simulink model "generic_20231123_1032"  (R2022b)
settings: Solver=ode45  StartTime=0.0  StopTime=50  RelTol=1e-3  EnableMultiTasking=on
model workspace (MAT data in the model file):
  A = 1
  Amplifier = -9.10007585438
  B = 1.19071237887
  K_d_yawrate = 0.231634180251
  K_dsteering = 5.24463953925
  k_speed = -0.570636497542
  k_stanley = 28.4909595466
  kd = -9.99955278144
  ki = 0.00519416981022
  kp = 9.99999979837
  path_curvature = 0
values from neighbouring files (symbols this model uses):
  brake_select = ones(length(speed), length(steering_angle))    [TwoDLook_uptable.m]
  curvature = 0.000:0.001:1    [TwoDLook_uptable.m]
  m = 1600    [MPCController1.m]    (also in MPCController2.m; MPC_Fmincon.m)
  speed = 0:0.1:100    [TwoDLook_uptable.m]
  steering_angle = -3.14/4:0.00628/4:3.14/4    [TwoDLook_uptable.m]
undefined symbols (not defined in the file or in its folder): DiscIntNeverNeededParam
libraries: CarMaker4SL x143, simulink x11, cstblocks x6, simulink_extras x4, autolibshared x1, mpcadaslib x1
(part 2 of 7)

== system generic_20231123_1032/CarMaker/IPG Vehicle/CarAndTrailer/Kinematics ==
  Sync_In : Inport
  Steer.IF : Inport  Port=2
  Kinematics : S-Function  FunctionName=CM_Sfun  Parameters='Kinematics'  SFunctionDeploymentMode=off  EnableBusSupport=off
  Sync_Out : Outport  VectorParamsAs1DForOutWhenUnconnected=off
  TireFL_In : Outport  Port=2  VectorParamsAs1DForOutWhenUnconnected=off
  TireFR_In : Outport  Port=3  VectorParamsAs1DForOutWhenUnconnected=off
  TireRL_In : Outport  Port=4  VectorParamsAs1DForOutWhenUnconnected=off
  TireRR_In : Outport  Port=5  VectorParamsAs1DForOutWhenUnconnected=off
  lSpring : Outport  Port=6  VectorParamsAs1DForOutWhenUnconnected=off
  vDamp : Outport  Port=7  VectorParamsAs1DForOutWhenUnconnected=off
  lStabi : Outport  Port=8  VectorParamsAs1DForOutWhenUnconnected=off
  lBuf : Outport  Port=9  VectorParamsAs1DForOutWhenUnconnected=off
  wires:
  Kinematics/9 -> lBuf/1
  Kinematics/8 -> lStabi/1
  Kinematics/2 -> TireFL_In/1
  Kinematics/3 -> TireFR_In/1
  Kinematics/4 -> TireRL_In/1
  Kinematics/5 -> TireRR_In/1
  Kinematics/6 -> lSpring/1
  Kinematics/7 -> vDamp/1
  Sync_In/1 -> Kinematics/1
  Kinematics/1 -> Sync_Out/1
  Steer.IF/1 -> Kinematics/2

== system generic_20231123_1032/CarMaker/IPG Vehicle/CarAndTrailer/Kinetics ==
  Sync_In : Inport
  Car.Virtual : Inport  Port=2
  Car.Aero : Inport  Port=3
  Car.Load : Inport  Port=4
  TireFL.Out : Inport  Port=5
  TireFR.Out : Inport  Port=6
  TireRL.Out : Inport  Port=7
  TireRR.Out : Inport  Port=8
  FSpring_ext : Inport  Port=9
  FDamp_ext : Inport  Port=10
  FStabi_ext : Inport  Port=11
  FBuf_ext : Inport  Port=12
  Bus Creator : BusCreator  Inputs=4
  Bus Creator1 : BusCreator  Inputs=12
  Bus Creator2 : BusCreator  Inputs=6
  Bus Creator3 : BusCreator  Inputs=6
  Bus Creator4 : BusCreator  Inputs=4
  Demux : Demux  Outputs=12
      settings: DisplayOption=none
  Demux1 : Demux  Outputs=6
      settings: DisplayOption=none
  Demux2 : Demux  Outputs=6
      settings: DisplayOption=none
  Demux3 : Demux
      settings: DisplayOption=none
  Demux4 : Demux
      settings: DisplayOption=none
  Kinetics : S-Function  FunctionName=CM_Sfun  Parameters='Kinetics'  SFunctionDeploymentMode=off  EnableBusSupport=off
  Sync_Out : Outport  VectorParamsAs1DForOutWhenUnconnected=off
  Trailer.Load : Outport  Port=2  VectorParamsAs1DForOutWhenUnconnected=off
  Car.Hitch : Outport  Port=3  VectorParamsAs1DForOutWhenUnconnected=off
  Car.Fr1 : Outport  Port=4  VectorParamsAs1DForOutWhenUnconnected=off
  Car.Trq_T2W : Outport  Port=5  VectorParamsAs1DForOutWhenUnconnected=off
  WheelCarrier.Misc : Outport  Port=6  VectorParamsAs1DForOutWhenUnconnected=off
  wires:
  FBuf_ext/1 -> Kinetics/12
  Sync_In/1 -> Kinetics/1
  Kinetics/1 -> Sync_Out/1
  Car.Aero/1 -> Kinetics/3
  Car.Virtual/1 -> Kinetics/2
  Bus Creator1/1 -> Trailer.Load/1
  Demux/1 -> Bus Creator1/1  "Trailer Load_0 mass"
  Demux/2 -> Bus Creator1/2  "Trailer Load_0 tx"
  Demux/3 -> Bus Creator1/3  "Trailer Load_0 ty"
  Demux/4 -> Bus Creator1/4  "Trailer Load_0 tz"
  Kinetics/2 -> Demux/1
  Demux/5 -> Bus Creator1/5  "Trailer Load_1 mass"
  Demux/6 -> Bus Creator1/6  "Trailer Load_1 tx"
  Demux/7 -> Bus Creator1/7  "Trailer Load_1 ty"
  Demux/8 -> Bus Creator1/8  "Trailer Load_1 tz"
  Demux/9 -> Bus Creator1/9  "Trailer Load_2 mass"
  Demux/10 -> Bus Creator1/10  "Trailer Load_2 tx"
  Demux/11 -> Bus Creator1/11  "Trailer Load_2 ty"
  Demux/12 -> Bus Creator1/12  "Trailer Load_2 tz"
  Demux1/1 -> Bus Creator2/1  "Car Hitch tx"
  Demux1/2 -> Bus Creator2/2  "Car Hitch ty"
  Demux1/3 -> Bus Creator2/3  "Car Hitch tz"
  Demux1/4 -> Bus Creator2/4  "Car Hitch vx"
  Demux1/5 -> Bus Creator2/5  "Car Hitch vy"
  Demux1/6 -> Bus Creator2/6  "Car Hitch vz"
  Kinetics/3 -> Demux1/1
  Bus Creator2/1 -> Car.Hitch/1
  Demux2/1 -> Bus Creator3/1  "Car Fr1 rx"
  Demux2/2 -> Bus Creator3/2  "Car Fr1 ry"
  Demux2/3 -> Bus Creator3/3  "Car Fr1 rz"
  Demux2/4 -> Bus Creator3/4  "Car Fr1 rvx"
  Demux2/5 -> Bus Creator3/5  "Car Fr1 rvy"
  Demux2/6 -> Bus Creator3/6  "Car Fr1 rvz"
  Bus Creator3/1 -> Car.Fr1/1
  Kinetics/4 -> Demux2/1
  Car.Load/1 -> Kinetics/4
  Demux3/1 -> Bus Creator4/1  "car Susp FL GenInert2"
  Demux3/2 -> Bus Creator4/2  "car Susp FR GenInert2"
  Demux3/3 -> Bus Creator4/3  "car Susp FL GenFrc2"
  Demux3/4 -> Bus Creator4/4  "car Susp FR GenFrc2"
  Bus Creator4/1 -> WheelCarrier.Misc/1
  Bus Creator/1 -> Car.Trq_T2W/1
  Demux4/4 -> Bus Creator/4  "Car Trq_T2WRR"
  Demux4/3 -> Bus Creator/3  "Car Trq_T2WRL"
  Demux4/2 -> Bus Creator/2  "Car Trq_T2WFR"
  Demux4/1 -> Bus Creator/1  "Car Trq_T2WFL"
  TireFL.Out/1 -> Kinetics/5
  TireFR.Out/1 -> Kinetics/6
  TireRL.Out/1 -> Kinetics/7
  TireRR.Out/1 -> Kinetics/8
  FSpring_ext/1 -> Kinetics/9
  FDamp_ext/1 -> Kinetics/10
  FStabi_ext/1 -> Kinetics/11
  Kinetics/6 -> Demux3/1
  Kinetics/5 -> Demux4/1

== system generic_20231123_1032/CarMaker/IPG Vehicle/CarAndTrailer/Steering ==
  note: When replacing the entire steering system,
      | be sure to disable the IPG steering model by using the steering
      | model 'Model Manager off' in the vehicle GUI.
  Sync_In : Inport
  VhclCtrl.Steering : Inport  Port=2
  Bus Creator1 : BusCreator  Inputs=16
  Bus Creator2 : BusCreator  Inputs=5
  Demux : Demux  Outputs=21
      settings: DisplayOption=none
  Steering : S-Function  FunctionName=CM_Sfun  Parameters='Steering'  SFunctionDeploymentMode=off  EnableBusSupport=off
  Terminator : Terminator
  Sync_Out : Outport  VectorParamsAs1DForOutWhenUnconnected=off
  Steer.IF : Outport  Port=2  VectorParamsAs1DForOutWhenUnconnected=off
  wires:
  Demux/21 -> Bus Creator2/5  "Steering IF R Inert"
  Demux/20 -> Bus Creator2/4  "Steering IF R Frc"
  Demux/19 -> Bus Creator2/3  "Steering IF L Inert"
  Demux/18 -> Bus Creator2/2  "Steering IF L Frc"
  Demux/17 -> Bus Creator2/1  "Steering IF SteerByTrq"
  Demux/16 -> Bus Creator1/16  "Steering IF R iSteer2q"
  Demux/15 -> Bus Creator1/15  "Steering IF R qpp"
  Demux/14 -> Bus Creator1/14  "Steering IF R qp"
  Demux/13 -> Bus Creator1/13  "Steering IF R q"
  Demux/12 -> Bus Creator1/12  "Steering IF L iSteer2q"
  Demux/11 -> Bus Creator1/11  "Steering IF L qpp"
  Demux/10 -> Bus Creator1/10  "Steering IF L qp"
  Demux/9 -> Bus Creator1/9  "Steering IF L q"
  Demux/8 -> Bus Creator1/8  "Steering IF AssistTrqPin"
  Demux/7 -> Bus Creator1/7  "Steering IF AssistTrqCol"
  Demux/6 -> Bus Creator1/6  "Steering IF AssistFrc"
  Demux/5 -> Bus Creator1/5  "Steering IF TrqStatic"
  Demux/4 -> Bus Creator1/4  "Steering IF Trq"
  Demux/3 -> Bus Creator1/3  "Steering IF AngAcc"
  Demux/2 -> Bus Creator1/2  "Steering IF AngVel"
  Demux/1 -> Bus Creator1/1  "Steering IF Ang"
  Bus Creator1/1 -> Steer.IF/1
  Steering/2 -> Demux/1
  Bus Creator2/1 -> Terminator/1  "Steer IF (in)"
  VhclCtrl.Steering/1 -> Steering/2
  Steering/1 -> Sync_Out/1
  Sync_In/1 -> Steering/1

== system generic_20231123_1032/CarMaker/IPG Vehicle/CarAndTrailer/Trailer ==
  Sync_In : Inport
  Trailer.Load : Inport  Port=2
  Car.Hitch : Inport  Port=3
  Car.Fr1 : Inport  Port=4
  Car.Trq_T2W : Inport  Port=5
  WheelCarrier.Misc : Inport  Port=6
  CreateBus Car.Hitch.FrcTrq : Subsystem
  CreateBus Vhcl.Motion : Subsystem
  CreateBus Vhcl.PoI : Subsystem
  CreateBus Vhcl.Steering : Subsystem
  CreateBus Vhcl.Wheel.FL : Subsystem
  CreateBus Vhcl.Wheel.FR : Subsystem
  CreateBus Vhcl.Wheel.RL : Subsystem
  CreateBus Vhcl.Wheel.RR : Subsystem
  Trailer : S-Function  FunctionName=CM_Sfun  Parameters='Trailer'  SFunctionDeploymentMode=off  EnableBusSupport=off
  Sync_Out : Outport  VectorParamsAs1DForOutWhenUnconnected=off
  Vhcl.Steering : Outport  Port=2  VectorParamsAs1DForOutWhenUnconnected=off
  Vhcl.Motion : Outport  Port=3  VectorParamsAs1DForOutWhenUnconnected=off
  Vhcl.PoI : Outport  Port=4  VectorParamsAs1DForOutWhenUnconnected=off
  Vhcl.Wheel.FL : Outport  Port=5  VectorParamsAs1DForOutWhenUnconnected=off
  Vhcl.Wheel.FR : Outport  Port=6  VectorParamsAs1DForOutWhenUnconnected=off
  Vhcl.Wheel.RL : Outport  Port=7  VectorParamsAs1DForOutWhenUnconnected=off
  Vhcl.Wheel.RR : Outport  Port=8  VectorParamsAs1DForOutWhenUnconnected=off
  Car.Hitch.FrcTrq : Outport  Port=9  VectorParamsAs1DForOutWhenUnconnected=off
  wires:
  Trailer/2 -> CreateBus Vhcl.Steering/1(In1)
  CreateBus Vhcl.Steering/1(Out1) -> Vhcl.Steering/1  "Vhcl.Steering"
  Trailer/3 -> CreateBus Vhcl.Motion/1(In1)
  Trailer/4 -> CreateBus Vhcl.PoI/1(In1)
  Trailer/5 -> CreateBus Vhcl.Wheel.FL/1(In1)
  Trailer/6 -> CreateBus Vhcl.Wheel.FR/1(In1)
  Trailer/7 -> CreateBus Vhcl.Wheel.RL/1(In1)
  Trailer/9 -> CreateBus Car.Hitch.FrcTrq/1(In1)
  Trailer/8 -> CreateBus Vhcl.Wheel.RR/1(In1)
  CreateBus Vhcl.Wheel.RR/1(Out1) -> Vhcl.Wheel.RR/1  "Vhcl.Wheel.RR"
  CreateBus Vhcl.Wheel.RL/1(Out1) -> Vhcl.Wheel.RL/1  "Vhcl.Wheel.RL"
  CreateBus Vhcl.Wheel.FR/1(Out1) -> Vhcl.Wheel.FR/1  "Vhcl.Wheel.FR"
  CreateBus Vhcl.Wheel.FL/1(Out1) -> Vhcl.Wheel.FL/1  "Vhcl.Wheel.FL"
  CreateBus Vhcl.PoI/1(Out1) -> Vhcl.PoI/1  "Vhcl.PoI"
  CreateBus Vhcl.Motion/1(Out1) -> Vhcl.Motion/1  "Vhcl.Motion"
  Car.Trq_T2W/1 -> Trailer/5
  WheelCarrier.Misc/1 -> Trailer/6
  CreateBus Car.Hitch.FrcTrq/1(Out1) -> Car.Hitch.FrcTrq/1  "Car.Hitch.FrcTrq"
  Car.Fr1/1 -> Trailer/4
  Car.Hitch/1 -> Trailer/3
  Trailer.Load/1 -> Trailer/2
  Trailer/1 -> Sync_Out/1
  Sync_In/1 -> Trailer/1

== system generic_20231123_1032/CarMaker/VehicleControl/CreateBus VhclCtrl/A*algoithm ==
  Bus Selector1 : BusSelector  OutputSignals=Path.tx,Path.ty
  Constant : Constant  Value=0
  Constant3 : Constant  Value=0
  Constant4 : Constant
  Gain : Gain  Gain=2
  MATLAB Function1 : MATLAB Function  TreatAsAtomicUnit=on
  Mux : Mux  Inputs=2
  Mux1 : Mux  Inputs=2
  Mux2 : Mux  Inputs=2
  Read CM Dict3 : CarMaker4SL/Read CM Dict  xname=Sensor.Radar.VehSensor_6.Obj0.Length  xsync=off  xstime=Continuous
  Read CM Dict4 : CarMaker4SL/Read CM Dict  xname=Traffic.T00.tx  xsync=off  xstime=Continuous
  Read CM Dict5 : CarMaker4SL/Read CM Dict  xname=Traffic.T00.ty  xsync=off  xstime=Continuous
  Read CM Dict6 : CarMaker4SL/Read CM Dict  xname=Sensor.Radar.VehSensor_6.Obj0.ProbObst  xsync=off  xstime=Continuous
  Read CM Dict7 : CarMaker4SL/Read CM Dict  xname=Sensor.Radar.VehSensor_6.Obj0.Width  xsync=off  xstime=Continuous
  Reshape : Reshape  OutputDimensionality=Customize  OutputDimensions=[1,2]
  Reshape1 : Reshape  OutputDimensionality=Customize  OutputDimensions=[1,2]
  Reshape2 : Reshape  OutputDimensionality=Customize  OutputDimensions=[1,2]
  Road Sensor1 : CarMaker4SL/Sensors/Road Sensor  xname=0  xstime=Continuous
      settings: SourceProductName=CarMaker4SL
  Subsystem : Subsystem  Commented=on
  Sum : Sum  Inputs=|++
  Switch : Switch  Criteria=u2 > Threshold  SaturateOnIntegerOverflow=off  InputSameDT=off
  Terminator : Terminator
  Terminator1 : Terminator
  Terminator2 : Terminator
  deviation : Outport
  pathX : Outport  Port=2
  pathY : Outport  Port=3
  wires:
  Constant4/1 -> Switch/1
  Road Sensor1/2 -> Bus Selector1/1
  Road Sensor1/1 -> Terminator/1
  Read CM Dict4/1 -> Mux1/1, Mux/1
  Constant3/1 -> Road Sensor1/1
  Read CM Dict6/1 -> Switch/2
  Constant/1 -> Switch/3
  Read CM Dict3/1 -> Gain/1
  Gain/1 -> Sum/1
  Read CM Dict5/1 -> Sum/2, Mux/2
  Mux2/1 -> Reshape/1
  Bus Selector1/1 -> Mux2/1  "<tx>"
  Bus Selector1/2 -> Mux2/2  "<ty>"
  Sum/1 -> Mux1/2
  Mux1/1 -> Reshape1/1
  Mux/1 -> Reshape2/1
  Reshape/1 -> MATLAB Function1/1(start)
  Reshape1/1 -> MATLAB Function1/2(target)
  Reshape2/1 -> MATLAB Function1/3(obstacles)
  MATLAB Function1/1(deviation) -> deviation/1
  MATLAB Function1/2(pathX) -> pathX/1
  MATLAB Function1/3(pathY) -> pathY/1
  Switch/1 -> Terminator1/1
  Read CM Dict7/1 -> Terminator2/1

== system generic_20231123_1032/CarMaker/VehicleControl/CreateBus VhclCtrl/MPC_steering_controllers ==
  Lateral_dev : Inport
  Dev_angle : Inport  Port=2
  Amplifyer : Gain  Gain=Amplifier
  Amplifyer1 : Gain  Gain=2
  Amplifyer2 : Gain  Gain=-3
  Bus Selector1 : BusSelector  OutputSignals=Path.tx,Path.ty,Path,Path.DevAng,Path.CurveXY
  Constant1 : Constant  Value=3
  Constant2 : Constant  Value=0
  Demux : Demux  Outputs=5
  Discrete-Time Integrator : DiscreteIntegrator  SampleTime=-1  ICPrevOutput=DiscIntNeverNeededParam  ICPrevScaledInput=DiscIntNeverNeededParam
  Gain : Gain  Gain=-1.6
  MATLAB System : MATLABSystem  Commented=on  System=MPCController  Nx=5  Nu=1  Ny=2  Np=20  Nc=10  T=0.01  lf=1.488  lr=1.487  Ccf=66900  Ccr=62700  m=1600  g=9.81  I=2986.624  x_dot=15  Q=diag( [ 2000, 0, 0, 10000, 0 ] )  R=5 * 10 ^ 5  Row=1000  umin=-0.6  umax=0.6  delta_umin=-0.06  delta_umax=0.06  ycmax=[ 0.2; 1000 ]  ycmin=[ -0.2; -1000 ]  SimulateUsing=Code generation
      mask Type: MPCController
      mask Display:
      | disp('MPCController');
      | port_label('input',1,'y_dot');
      | port_label('input',2,'phi');
      | port_label('input',3,'phi_dot');
      | port_label('input',4,'Y');
      | port_label('input',5,'X');
      | port_label('output',1,'delta_f');
      | port_label('output',2,'state_k1');
  Multiport Switch : MultiPortSwitch  SaturateOnIntegerOverflow=off  InputSameDT=off
  Mux1 : Mux  Inputs=5
  Mux3 : Mux  Inputs=1
  Product : Product
  Radians to Degrees : simulink_extras/Transformations/Radians to Degrees
  Radians to Degrees1 : simulink_extras/Transformations/Radians to Degrees
  Read CM Dict : CarMaker4SL/Read CM Dict  xname=Sensor.Road.VehSensor_0.Path.DevAng  xsync=off  xstime=Continuous
  Read CM Dict1 : CarMaker4SL/Read CM Dict  xname=Car.Road.Path.DevDist  xsync=off  xstime=Continuous
  Read CM Dict8 : CarMaker4SL/Read CM Dict  xname=Vhcl.v  xsync=off  xstime=Continuous
  Road Sensor1 : CarMaker4SL/Sensors/Road Sensor  xname=0  xstime=Continuous
      settings: SourceProductName=CarMaker4SL
  S-Function1 : S-Function  FunctionName=MPCController1  SFunctionDeploymentMode=off  EnableBusSupport=off
  Scope : Scope
  Sign : Signum
  State_space_system_variables : Subsystem
  Subsystem : Subsystem  Commented=on
  Sum : Sum  Inputs=|+++
  Terminator : Terminator
  Terminator1 : Terminator  Commented=on
  Terminator2 : Terminator
  Terminator3 : Terminator
  Traditional_MPC : Subsystem
  steering : Outport
  wires:
  Constant2/1 -> Road Sensor1/1
  Demux/1 -> MATLAB System/4
  Bus Selector1/5 -> Product/2  "<CurveXY>"
  Bus Selector1/3 -> Terminator1/1  "<Path>"
  Road Sensor1/1 -> Terminator/1
  Road Sensor1/2 -> Bus Selector1/1
  Mux3/1 -> S-Function1/1, Demux/1
  Read CM Dict8/1 -> Product/1
  Bus Selector1/1 -> State_space_system_variables/3(X_ref_m), Mux1/5  "<tx>"
  Bus Selector1/2 -> State_space_system_variables/2(Y_ref_m), Mux1/4  "<ty>"
  Product/1 -> Discrete-Time Integrator/1, Radians to Degrees1/1
  Discrete-Time Integrator/1 -> Radians to Degrees/1
  Radians to Degrees/1 -> State_space_system_variables/1(Yaw_ref_deg), Mux1/2
  Constant1/1 -> Multiport Switch/1
  Radians to Degrees1/1 -> Mux1/3
  State_space_system_variables/1(x) -> Mux3/1
  Demux/5 -> MATLAB System/3
  Demux/3 -> MATLAB System/1
  State_space_system_variables/2(Lateral_velocity) -> Mux1/1
  Read CM Dict/1 -> Amplifyer/1
  Mux1/1 -> Terminator2/1  "u"
  Read CM Dict1/1 -> Amplifyer1/1
  Amplifyer/1 -> Amplifyer2/1  "Dev_angle"
  Demux/2 -> MATLAB System/5
  Demux/4 -> MATLAB System/2
  Amplifyer1/1 -> Traditional_MPC/1(Lateral_deviation)  "Dev_angle"
  Amplifyer2/1 -> Traditional_MPC/2(Dev_angle)  "Dev_angle"
  MATLAB System/1 -> Multiport Switch/3
  Multiport Switch/1 -> steering/1
  MATLAB System/2 -> Terminator3/1
  S-Function1/1 -> Sign/1, Sum/1, Multiport Switch/2
  Traditional_MPC/1(steering_cmd) -> Multiport Switch/4
  Sum/1 -> Scope/1
  Traditional_MPC/2(Heading_correction) -> Sum/2
  Sign/1 -> Gain/1
  Gain/1 -> Sum/3

== system generic_20231123_1032/CarMaker/VehicleControl/CreateBus VhclCtrl/PID steering controller ==
  Lateral_error : Inport
  Add : Sum  Inputs=+++
  Dervative : Subsystem
  Discrete-Time Integrator : DiscreteIntegrator  SampleTime=-1  ICPrevOutput=DiscIntNeverNeededParam  ICPrevScaledInput=DiscIntNeverNeededParam
  Gain : Gain  Gain=1.1
  Gain1 : Gain  Gain=0.9
  steering_cmd : Outport
  wires:
  Lateral_error/1 -> Gain1/1, Gain/1, Dervative/1(Error)
  Discrete-Time Integrator/1 -> Add/1
  Gain1/1 -> Discrete-Time Integrator/1
  Gain/1 -> Add/2
  Add/1 -> steering_cmd/1
  Dervative/1(Dervative term) -> Add/3

== system generic_20231123_1032/CarMaker/VehicleControl/CreateBus VhclCtrl/Smoothing ==
  Signal_In : Inport
  Add : Sum  Inputs=++++
  Delay : Delay  InitialCondition=0.1
  Delay1 : Delay  DelayLength=4  InitialCondition=0.1
  Delay2 : Delay  DelayLength=5  InitialCondition=0.1
  Gain : Gain  Gain=0.35
  Gain1 : Gain  Gain=0.25
  Gain2 : Gain  Gain=0.25
  Gain3 : Gain  Gain=0.15
  Signal_Out : Outport  VectorParamsAs1DForOutWhenUnconnected=off
  wires:
  Gain1/1 -> Add/2
  Signal_In/1 -> Gain/1
  Delay/1 -> Gain1/1
  Gain/1 -> Add/1
  Delay1/1 -> Gain2/1
  Add/1 -> Delay2/1, Delay1/1, Delay/1, Signal_Out/1
  Gain2/1 -> Add/3
  Delay2/1 -> Gain3/1
  Gain3/1 -> Add/4

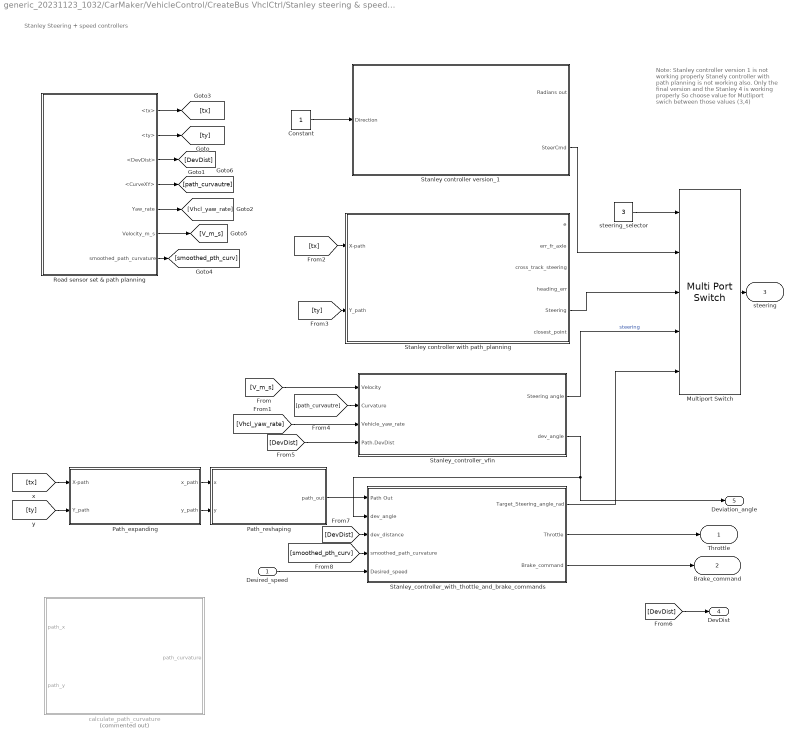
== system generic_20231123_1032/CarMaker/VehicleControl/CreateBus VhclCtrl/Stanley steering & speed//Brake controller ==
  note: Note:
      | Stanley controller version 1 is not working properly
      | Stanely controller with path planning is not working also.
      | Only the final version and the Stanley 4 is working properly
      | So choose value for Mutliport swich between those values (3,4)
  note: Stanley Steering + speed controllers
  Desired_speed : Inport
  " Path_expanding" : Subsystem
  Constant : Constant
  Multiport Switch : MultiPortSwitch  Inputs=4  SaturateOnIntegerOverflow=off  InputSameDT=off
  Path_reshaping : MATLAB Function  TreatAsAtomicUnit=on
  Road sensor set & path planning : Subsystem  Variant=on  VariantControlMode=label  VariantControl=Choice  LabelModeActiveChoice=Choice
  Stanley controller version_1 : Subsystem  Variant=on  VariantControlMode=label  VariantControl=Choice  LabelModeActiveChoice=Choice
  Stanley controller with path_planning : Subsystem  Variant=on  VariantControlMode=label  VariantControl=Choice  LabelModeActiveChoice=Choice
  Stanley_controller_vfin : Subsystem  Variant=on  VariantControlMode=label  VariantControl=Choice  LabelModeActiveChoice=Choice
  Stanley_controller_with_thottle_and_brake_commands : Subsystem
  calculate_path_curvature : Subsystem  Commented=on  Variant=on  VariantControlMode=label  VariantControl=Choice  LabelModeActiveChoice=Choice
  steering_selector : Constant  Value=3
  Throttle : Outport
  Brake_command : Outport  Port=2
  steering : Outport  Port=3
  DevDist : Outport  Port=4
  Deviation_angle : Outport  Port=5
  wires:
  [tx] -> " Path_expanding"/1(X-path)
  [ty] -> " Path_expanding"/2(Y_path)
  [tx] -> Stanley controller with path_planning/1(X-path)
  [ty] -> Stanley controller with path_planning/2(Y_path)
  Road sensor set & path planning/1(<tx>) -> [tx]
  Road sensor set & path planning/2(<ty>) -> [ty]
  Road sensor set & path planning/3(<DevDist>) -> [DevDist]
  Road sensor set & path planning/4(<CurveXY>) -> [path_curvautre]
  Road sensor set & path planning/5(Yaw_rate) -> [Vhcl_yaw_rate]
  [path_curvautre] -> Stanley_controller_vfin/2(Curvature)
  Stanley_controller_vfin/1(Steering angle) -> Multiport Switch/4  "steering"
  Constant/1 -> Stanley controller version_1/1(Direction)
  steering_selector/1 -> Multiport Switch/1
  Stanley controller version_1/2(SteerCmd) -> Multiport Switch/2
  Stanley controller with path_planning/5(Steering) -> Multiport Switch/3
  Path_reshaping/1(path_out) -> Stanley_controller_with_thottle_and_brake_commands/1(Path Out)
  Stanley_controller_vfin/2(dev_angle) -> Deviation_angle/1, Stanley_controller_with_thottle_and_brake_commands/2(dev_angle)
  " Path_expanding"/1(x_path) -> Path_reshaping/1(x)
  " Path_expanding"/2(y_path) -> Path_reshaping/2(y)
  Stanley_controller_with_thottle_and_brake_commands/2(Throttle) -> Throttle/1
  Stanley_controller_with_thottle_and_brake_commands/3(Brake_command) -> Brake_command/1
  Stanley_controller_with_thottle_and_brake_commands/1(Target_Steering_angle_rad) -> Multiport Switch/5
  [V_m_s] -> Stanley_controller_vfin/1(Velocity)
  [Vhcl_yaw_rate] -> Stanley_controller_vfin/3(Vehicle_yaw_rate)
  [DevDist] -> Stanley_controller_vfin/4(Path.DevDist)
  Road sensor set & path planning/6(Velocity_m_s) -> [V_m_s]
  [DevDist] -> DevDist/1
  Multiport Switch/1 -> steering/1
  [DevDist] -> Stanley_controller_with_thottle_and_brake_commands/3(dev_distance)
  Road sensor set & path planning/7(smoothed_path_curvature) -> [smoothed_pth_curv]
  [smoothed_pth_curv] -> Stanley_controller_with_thottle_and_brake_commands/4(smoothed_path_curvature)
  Desired_speed/1 -> Stanley_controller_with_thottle_and_brake_commands/5(Desired_speed)

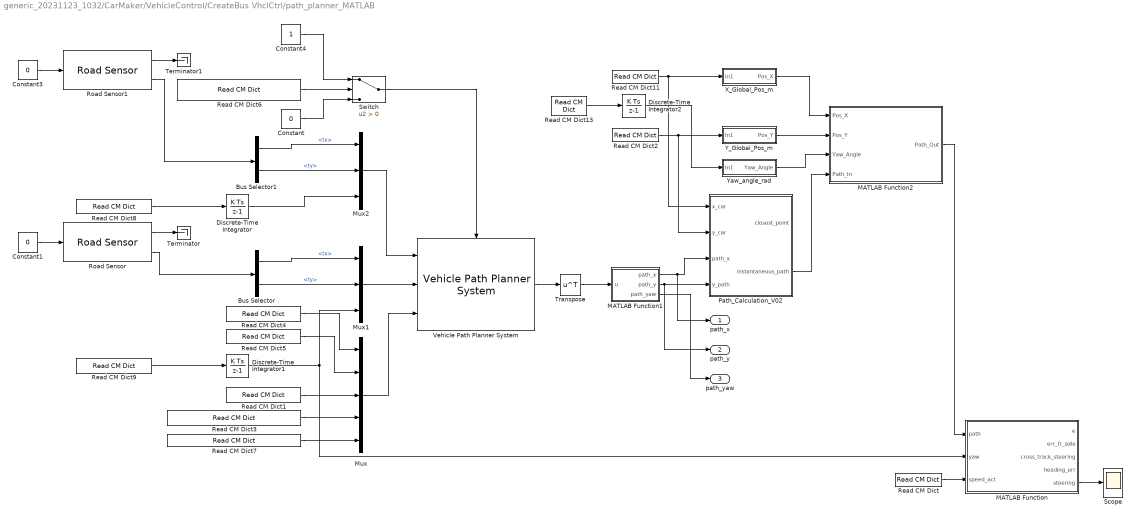
== system generic_20231123_1032/CarMaker/VehicleControl/CreateBus VhclCtrl/path_planner_MATLAB ==
  Bus Selector : BusSelector  OutputSignals=Path.tx,Path.ty
  Bus Selector1 : BusSelector  OutputSignals=Path.tx,Path.ty
  Constant : Constant  Value=0
  Constant1 : Constant  Value=0
  Constant3 : Constant  Value=0
  Constant4 : Constant
  Discrete-Time Integrator : DiscreteIntegrator  SampleTime=-1  ICPrevOutput=DiscIntNeverNeededParam  ICPrevScaledInput=DiscIntNeverNeededParam
  Discrete-Time Integrator1 : DiscreteIntegrator  SampleTime=-1  ICPrevOutput=DiscIntNeverNeededParam  ICPrevScaledInput=DiscIntNeverNeededParam
  Discrete-Time Integrator2 : DiscreteIntegrator  SampleTime=-1  ICPrevOutput=DiscIntNeverNeededParam  ICPrevScaledInput=DiscIntNeverNeededParam
  MATLAB Function : MATLAB Function  TreatAsAtomicUnit=on
  MATLAB Function1 : MATLAB Function  TreatAsAtomicUnit=on
  MATLAB Function2 : MATLAB Function  TreatAsAtomicUnit=on
  Mux : Mux  Inputs=5
  Mux1 : Mux  Inputs=3
  Mux2 : Mux  Inputs=3
  Path_Calculation_V02 : MATLAB Function  TreatAsAtomicUnit=on
  Read CM Dict : CarMaker4SL/Read CM Dict  xname=Vhcl.v  xsync=off  xstime=Continuous
  Read CM Dict1 : CarMaker4SL/Read CM Dict  xname=Traffic.T00.rz  xsync=off  xstime=Continuous
  Read CM Dict11 : CarMaker4SL/Read CM Dict  xname=Car.Gen.tx  xsync=off  xstime=Continuous
  Read CM Dict13 : CarMaker4SL/Read CM Dict  xname=Car.YawRate  xsync=off  xstime=Continuous
  Read CM Dict2 : CarMaker4SL/Read CM Dict  xname=Car.Gen.ty  xsync=off  xstime=Continuous
  Read CM Dict3 : CarMaker4SL/Read CM Dict  xname=Sensor.Radar.VehSensor_6.Obj0.Length  xsync=off  xstime=Continuous
  Read CM Dict4 : CarMaker4SL/Read CM Dict  xname=Traffic.T00.tx  xsync=off  xstime=Continuous
  Read CM Dict5 : CarMaker4SL/Read CM Dict  xname=Traffic.T00.ty  xsync=off  xstime=Continuous
  Read CM Dict6 : CarMaker4SL/Read CM Dict  xname=Sensor.Radar.VehSensor_6.Obj0.ProbObst  xsync=off  xstime=Continuous
  Read CM Dict7 : CarMaker4SL/Read CM Dict  xname=Sensor.Radar.VehSensor_6.Obj0.Width  xsync=off  xstime=Continuous
  Read CM Dict8 : CarMaker4SL/Read CM Dict  xname=Car.YawRate  xsync=off  xstime=Continuous
  Read CM Dict9 : CarMaker4SL/Read CM Dict  xname=Car.YawRate  xsync=off  xstime=Continuous
  Road Sensor : CarMaker4SL/Sensors/Road Sensor  xname=0  xstime=Continuous
      settings: SourceProductName=CarMaker4SL
  Road Sensor1 : CarMaker4SL/Sensors/Road Sensor  xname=0  xstime=Continuous
      settings: SourceProductName=CarMaker4SL
  Scope : Scope
  Switch : Switch  Criteria=u2 > Threshold  SaturateOnIntegerOverflow=off  InputSameDT=off
  Terminator : Terminator
  Terminator1 : Terminator
  Transpose : Math  Operator=transpose
  Vehicle Path Planner System : mpcadaslib/Vehicle Path Planner System  egoLength=4.7  egoWidth=1.8  wheelbase=2.8  dist2Center=1.4  numObs=1  obsMat=zeros(1,5)  obs_ext=on  minDist=1  Ts=1  pPlanning=20  v_range=[-20,30]  v_ext=off  steer_range=[-pi/4,pi/4]  steer_ext=off  suboptimal=off  maxiter=200  output_exitflag=off
      settings: LibrarySourceBlock=mpclib/Automated Driving/Vehicle Path Planner System
  X_Global_Pos_m : Subsystem
  Y_Global_Pos_m : Subsystem
  Yaw_angle_rad : Subsystem
  path_x : Outport
  path_y : Outport  Port=2
  path_yaw : Outport  Port=3
  wires:
  Constant3/1 -> Road Sensor1/1
  Mux1/1 -> Vehicle Path Planner System/2
  Road Sensor/1 -> Terminator/1
  Road Sensor1/1 -> Terminator1/1
  Constant1/1 -> Road Sensor/1
  Bus Selector1/2 -> Mux2/2  "<ty>"
  Read CM Dict9/1 -> Discrete-Time Integrator1/1
  Road Sensor/2 -> Bus Selector/1
  Road Sensor1/2 -> Bus Selector1/1
  Read CM Dict8/1 -> Discrete-Time Integrator/1
  MATLAB Function2/1(Path_Out) -> MATLAB Function/1(path)
  Constant4/1 -> Switch/1
  Read CM Dict6/1 -> Switch/2
  Constant/1 -> Switch/3
  MATLAB Function1/1(path_x) -> Path_Calculation_V02/3(path_x), path_x/1
  Bus Selector1/1 -> Mux2/1  "<tx>"
  Discrete-Time Integrator/1 -> Mux2/3
  Bus Selector/1 -> Mux1/1  "<tx>"
  Bus Selector/2 -> Mux1/2  "<ty>"
  X_Global_Pos_m/1(Pos_X) -> MATLAB Function2/1(Pos_X)
  Read CM Dict4/1 -> Mux/1
  Read CM Dict5/1 -> Mux/2
  Read CM Dict11/1 -> Path_Calculation_V02/1(x_car), X_Global_Pos_m/1(In1)
  Discrete-Time Integrator1/1 -> MATLAB Function/2(yaw), Mux1/3
  Read CM Dict1/1 -> Mux/3
  Read CM Dict3/1 -> Mux/4
  Y_Global_Pos_m/1(Pos_Y) -> MATLAB Function2/2(Pos_Y)
  Read CM Dict7/1 -> Mux/5
  Transpose/1 -> MATLAB Function1/1(u)
  Switch/1 -> Vehicle Path Planner System/Enable
  Mux2/1 -> Vehicle Path Planner System/1
  Mux/1 -> Vehicle Path Planner System/3
  Vehicle Path Planner System/1 -> Transpose/1
  Read CM Dict13/1 -> Discrete-Time Integrator2/1
  Discrete-Time Integrator2/1 -> Yaw_angle_rad/1(In1)
  Read CM Dict2/1 -> Path_Calculation_V02/2(y_car), Y_Global_Pos_m/1(In1)
  MATLAB Function/5(steering) -> Scope/1
  MATLAB Function1/2(path_y) -> path_y/1, Path_Calculation_V02/4(y_path)
  MATLAB Function1/3(path_yaw) -> path_yaw/1
  Yaw_angle_rad/1(Yaw_Angle) -> MATLAB Function2/3(Yaw_Angle)
  Path_Calculation_V02/2(instantaneous_path) -> MATLAB Function2/4(Path_In)
  Read CM Dict/1 -> MATLAB Function/3(speed_act)

== system generic_20231123_1032/CarMaker/VehicleControl/Subsystem/ Path_expanding ==
  X-path : Inport
  Y_path : Inport  Port=2
  Delay1 : Delay  DelayLength=9
  Delay10 : Delay  DelayLength=3
  Delay11 : Delay  DelayLength=4
  Delay13 : Delay  DelayLength=6
  Delay14 : Delay  DelayLength=7
  Delay15 : Delay  DelayLength=8
  Delay25 : Delay  DelayLength=7
  Delay26 : Delay  DelayLength=8
  Delay3 : Delay  DelayLength=9
  Delay37 : Delay  DelayLength=1
  Delay38 : Delay
  Delay4 : Delay  DelayLength=1
  Delay5 : Delay  DelayLength=3
  Delay6 : Delay  DelayLength=4
  Delay8 : Delay  DelayLength=6
  Delay9 : Delay
  Mux1 : Mux  Inputs=9
  Mux2 : Mux  Inputs=9
  Reshape1 : Reshape  OutputDimensionality=Customize  OutputDimensions=[1,9]
  Reshape2 : Reshape  OutputDimensionality=Customize  OutputDimensions=[1,9]
  x_path : Outport
  y_path : Outport  Port=2
  wires:
  X-path/1 -> Mux2/1, Delay38/1, Delay37/1, Delay5/1, Delay6/1, Delay8/1, Delay25/1, Delay26/1, Delay3/1
  Delay25/1 -> Mux2/7
  Y_path/1 -> Mux1/1, Delay4/1, Delay9/1, Delay10/1, Delay11/1, Delay13/1, Delay14/1, Delay15/1, Delay1/1
  Delay5/1 -> Mux2/4
  Delay37/1 -> Mux2/2
  Delay6/1 -> Mux2/5
  Delay38/1 -> Mux2/3
  Delay8/1 -> Mux2/6
  Delay26/1 -> Mux2/8
  Mux1/1 -> Reshape1/1
  Delay1/1 -> Mux1/9
  Delay15/1 -> Mux1/8
  Reshape1/1 -> y_path/1
  Delay4/1 -> Mux1/2
  Delay9/1 -> Mux1/3
  Delay10/1 -> Mux1/4
  Delay11/1 -> Mux1/5
  Delay13/1 -> Mux1/6
  Reshape2/1 -> x_path/1
  Delay14/1 -> Mux1/7
  Mux2/1 -> Reshape2/1
  Delay3/1 -> Mux2/9

== system generic_20231123_1032/CarMaker/VehicleControl/Subsystem/PID steering controller ==
  Lateral_error : Inport
  Add : Sum  Inputs=+++
  Derivative : Derivative
  Discrete-Time Integrator : DiscreteIntegrator  SampleTime=-1  ICPrevOutput=DiscIntNeverNeededParam  ICPrevScaledInput=DiscIntNeverNeededParam
  Gain : Gain  Gain=0.6
  Gain1 : Gain  Gain=0.9
  Gain2 : Gain  Gain=0.4
  steering_cmd : Outport
  wires:
  Lateral_error/1 -> Gain1/1, Gain/1, Gain2/1
  Discrete-Time Integrator/1 -> Add/1
  Gain2/1 -> Derivative/1
  Gain1/1 -> Discrete-Time Integrator/1
  Gain/1 -> Add/2
  Derivative/1 -> Add/3
  Add/1 -> steering_cmd/1

== system generic_20231123_1032/CarMaker/VehicleControl/Subsystem/Subsystem3 ==
  AND : Logic  IconShape=distinctive  AllPortsSameDT=off  OutDataTypeStr=boolean
  AND1 : Logic  IconShape=distinctive  AllPortsSameDT=off  OutDataTypeStr=boolean
  Clock{,2..6} (6 alike) : Clock
  Compare To Constant : simulink/Logic and Bit Operations/Compare To Constant  relop=>=  const=8  OutDataTypeStr=boolean
  Compare To Constant2 : simulink/Logic and Bit Operations/Compare To Constant  relop=>=  const=0.05  OutDataTypeStr=boolean
  Compare To Constant3 : simulink/Logic and Bit Operations/Compare To Constant  relop=<  const=4  OutDataTypeStr=boolean
  Compare To Constant5 : simulink/Logic and Bit Operations/Compare To Constant  relop=>  const=4  OutDataTypeStr=boolean
  Compare To Constant6 : simulink/Logic and Bit Operations/Compare To Constant  relop=<  const=8  OutDataTypeStr=boolean
  Gain : Gain  Gain=1.95
  Gain2 : Gain  Gain=2
  Gain4 : Gain  Gain=2.4
  Sum3 : Sum  Inputs=|+++
  Out1 : Outport
  Out2 : Outport  Port=2
  wires:
  Clock4/1 -> Out2/1
  Clock5/1 -> Compare To Constant5/1
  Clock6/1 -> Compare To Constant6/1
  Compare To Constant6/1 -> AND1/2
  Clock2/1 -> Compare To Constant2/1
  Clock3/1 -> Compare To Constant3/1
  Clock/1 -> Compare To Constant/1
  Compare To Constant5/1 -> AND1/1
  AND1/1 -> Gain4/1
  Compare To Constant2/1 -> AND/1
  Compare To Constant3/1 -> AND/2
  Compare To Constant/1 -> Gain/1
  AND/1 -> Gain2/1
  Gain/1 -> Sum3/2
  Gain4/1 -> Sum3/3
  Gain2/1 -> Sum3/1
  Sum3/1 -> Out1/1

== system generic_20231123_1032/CarMaker/VehicleControl/Subsystem1/Cross_track_error_calcuation ==
  y_path : Inport
  x_path : Inport  Port=2
  Cross_track_error_calcuation : MATLAB Function  TreatAsAtomicUnit=on
  Delay : Delay  DelayLength=1
  Delay1 : Delay  DelayLength=1
  Gain1 : Gain  Gain=-1
  Read CM Dict12 : CarMaker4SL/Read CM Dict  xname=Car.Gen.ty  xsync=off  xstime=Continuous
  Read CM Dict8 : CarMaker4SL/Read CM Dict  xname=Car.Gen.tx  xsync=off  xstime=Continuous
  cte : Outport
  denominator : Outport  Port=2
  wires:
  Read CM Dict12/1 -> Cross_track_error_calcuation/2(y_vehicle)
  x_path/1 -> Cross_track_error_calcuation/5(x2), Delay1/1
  y_path/1 -> Cross_track_error_calcuation/6(y2), Delay/1
  Cross_track_error_calcuation/2(denominator) -> denominator/1
  Read CM Dict8/1 -> Cross_track_error_calcuation/1(x_vehicle)
  Delay1/1 -> Cross_track_error_calcuation/3(x_point)
  Delay/1 -> Cross_track_error_calcuation/4(y_point)
  Cross_track_error_calcuation/1(cte) -> Gain1/1
  Gain1/1 -> cte/1

== system generic_20231123_1032/CarMaker/VehicleControl/Subsystem1/Obstacle_data_gathering ==
  y_dev : Inport
  Constant5 : Constant  Value=1.97
  Gain2 : Gain  Gain=-1
  MATLAB Function6 : MATLAB Function  TreatAsAtomicUnit=on
  MATLAB Function8 : MATLAB Function  TreatAsAtomicUnit=on
  Read CM Dict : CarMaker4SL/Read CM Dict  xname=Sensor.Object.VehSensor_5.relvTgt.NearPnt.ds.y  xsync=off  xstime=Continuous
  Read CM Dict1 : CarMaker4SL/Read CM Dict  xname=Car.Road.Path.DevDist  xsync=off  xstime=Continuous
  Read CM Dict11 : CarMaker4SL/Read CM Dict  xname=Sensor.Object.RadarL.relvTgt.NearPnt.ds.y  xsync=off  xstime=Continuous
  Read CM Dict13 : CarMaker4SL/Read CM Dict  xname=Sensor.Object.RadarL.Obj.T00.RefPnt.ds.x  xsync=off  xstime=Continuous
  Read CM Dict16 : CarMaker4SL/Read CM Dict  xname=Sensor.Object.VehSensor_4.relvTgt.NearPnt.ds.y  xsync=off  xstime=Continuous
  Read CM Dict17 : CarMaker4SL/Read CM Dict  xname=Sensor.Object.RadarL.relvTgt.NearPnt.ds.x  xsync=off  xstime=Continuous
  Scope : Scope  NumInputPorts=2
  Subsystem : Subsystem
  y_added : Outport
  Signal_In : Outport  Port=2
  wires:
  y_dev/1 -> MATLAB Function8/1(y_dev)
  Read CM Dict17/1 -> MATLAB Function6/7(x_distance_obj)
  Read CM Dict1/1 -> MATLAB Function6/1(path_dev)
  Constant5/1 -> MATLAB Function6/2(y_dev)
  Read CM Dict13/1 -> Scope/1, MATLAB Function8/3(distance), MATLAB Function6/6(distance)
  Read CM Dict11/1 -> MATLAB Function6/4(y_error_2)
  Read CM Dict16/1 -> MATLAB Function6/3(y_error3)
  Read CM Dict/1 -> MATLAB Function6/5(y_error), MATLAB Function8/2(data)
  MATLAB Function8/1(y_added) -> y_added/1
  MATLAB Function6/1(error) -> Gain2/1, Scope/2
  Gain2/1 -> Subsystem/1(In1)
  Subsystem/1(Signal_In) -> Signal_In/1

== system generic_20231123_1032/CarMaker/VehicleControl/Subsystem1/calculate_cross_track_error ==
  Acos : Trigonometry  Operator=asin
  Bus Selector2 : BusSelector  OutputSignals=Path.tx,Path.ty,Path.DevAng
  Constant : Constant  Value=0.2
  Constant1 : Constant  Value=0.2
  Constant3 : Constant  Value=0
  Delay2 : Delay  DelayLength=1
  Delay3 : Delay  DelayLength=1
  Divide : Product  Inputs=/*
  Read CM Dict14 : CarMaker4SL/Read CM Dict  xname=Car.Gen.ty  xsync=off  xstime=Continuous
  Read CM Dict15 : CarMaker4SL/Read CM Dict  xname=Car.Gen.tx  xsync=off  xstime=Continuous
  Read CM Dict6 : CarMaker4SL/Read CM Dict  Commented=on  xname=Car.Road.Path.DevDist  xsync=off  xstime=Continuous
  Road Sensor2 : CarMaker4SL/Sensors/Road Sensor  xname=0  xstime=Continuous
      settings: SourceProductName=CarMaker4SL
  Scope : Scope  Commented=on  NumInputPorts=3
  Scope1 : Scope  NumInputPorts=2
  Sqrt : Sqrt
  Sqrt1 : Sqrt
  Square{,1..3} (4 alike) : Math  Operator=square
  Sum{1..2,4,6..7} (5 alike) : Sum  Inputs=|+-
  Sum3 : Sum  Inputs=|++
  Sum5 : Sum  Inputs=|++
  Sum8 : Sum  Inputs=|++
  Terminator{,1..3} (4 alike) : Terminator
  calculate_cross_track_error : MATLAB Function  Commented=on  TreatAsAtomicUnit=on
  cte : Outport
  denominator : Outport  Port=2
  wires:
  ? -> Terminator2/1  "<Path>"
  calculate_cross_track_error/2(slope) -> Scope/2, denominator/1
  Constant3/1 -> Road Sensor2/1
  Bus Selector2/2 -> Sum3/1, calculate_cross_track_error/4(y_point), Sum6/2, Delay2/1  "<ty>"
  Road Sensor2/1 -> Terminator3/1
  Road Sensor2/2 -> Bus Selector2/1
  Bus Selector2/1 -> Sum7/2, Sum2/1, calculate_cross_track_error/3(x_point), Delay3/1  "<tx>"
  Bus Selector2/3 -> Scope1/2, Terminator/1  "<DevAng>"
  ? -> Terminator1/1  "<CurveXY>"
  Read CM Dict15/1 -> Sum1/2, calculate_cross_track_error/1(x_vehicle), Sum7/1
  calculate_cross_track_error/1(cte) -> Scope/1, cte/1
  Read CM Dict6/1 -> Scope/3
  Delay2/1 -> calculate_cross_track_error/6(y2)
  Delay3/1 -> calculate_cross_track_error/5(x2)
  Constant/1 -> Sum2/2
  Constant1/1 -> Sum3/2
  Sum2/1 -> Sum1/1
  Sum3/1 -> Sum4/1
  Sum4/1 -> Square/1
  Sum1/1 -> Square1/1
  Square/1 -> Sum5/2
  Square1/1 -> Sum5/1
  Sum5/1 -> Sqrt/1
  Square2/1 -> Sum8/2
  Sum7/1 -> Square2/1
  Sum8/1 -> Sqrt1/1
  Square3/1 -> Sum8/1
  Sum6/1 -> Square3/1
  Read CM Dict14/1 -> calculate_cross_track_error/2(y_vehicle), Sum4/2, Sum6/1
  Sqrt/1 -> Divide/1
  Sqrt1/1 -> Divide/2
  Divide/1 -> Acos/1
  Acos/1 -> Scope1/1

== system generic_20231123_1032/CarMaker/IPG Vehicle/CarAndTrailer/CarAndTrailerUpd/CreateBus Brake.IF.In ==
  In : Inport
  BusCreator : BusCreator  Inputs=9
  Demux : Demux  Outputs=9
      settings: DisplayOption=none
  Out : Outport  VectorParamsAs1DForOutWhenUnconnected=off
  wires:
  Demux/9 -> BusCreator/9  "Brake IF Trq_Reg RR"
  Demux/8 -> BusCreator/8  "Brake IF Trq_Reg RL"
  Demux/7 -> BusCreator/7  "Brake IF Trq_Reg FR"
  Demux/6 -> BusCreator/6  "Brake IF Trq_Reg FL"
  Demux/5 -> BusCreator/5  "Brake IF Trq_Reg_max RR"
  Demux/4 -> BusCreator/4  "Brake IF Trq_Reg_max RL"
  Demux/3 -> BusCreator/3  "Brake IF Trq_Reg_max FR"
  Demux/2 -> BusCreator/2  "Brake IF Trq_Reg_max FL"
  Demux/1 -> BusCreator/1  "Brake IF T_env"
  BusCreator/1 -> Out/1
  In/1 -> Demux/1

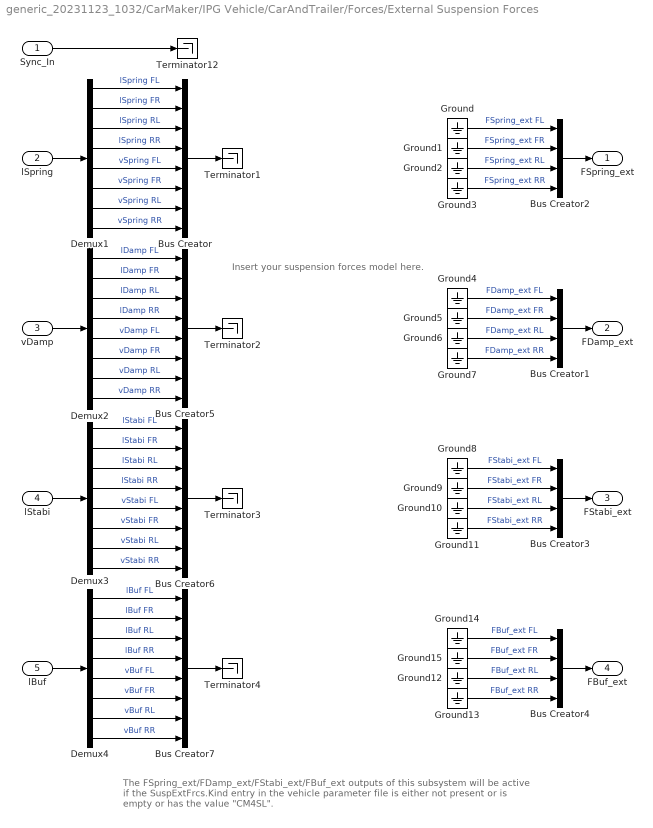
== system generic_20231123_1032/CarMaker/IPG Vehicle/CarAndTrailer/Forces/External Suspension Forces ==
  note: The FSpring_ext/FDamp_ext/FStabi_ext/FBuf_ext outputs of this subsystem will be
      | active if the SuspExtFrcs.Kind entry in the vehicle parameter file
      | is either not present or is empty or has the value "CM4SL".
  note: Insert your suspension forces model here.
  Sync_In : Inport
  lSpring : Inport  Port=2
  vDamp : Inport  Port=3
  lStabi : Inport  Port=4
  lBuf : Inport  Port=5
  Bus Creator{,5..7} (4 alike) : BusCreator  Inputs=8
  Bus Creator{1..4} (4 alike) : BusCreator  Inputs=4
  Demux{1..4} (4 alike) : Demux  Outputs=8
      settings: DisplayOption=none
  Ground{,1..15} (16 alike) : Ground
  Terminator{1..4,12} (5 alike) : Terminator
  FSpring_ext : Outport  VectorParamsAs1DForOutWhenUnconnected=off
  FDamp_ext : Outport  Port=2  VectorParamsAs1DForOutWhenUnconnected=off
  FStabi_ext : Outport  Port=3  VectorParamsAs1DForOutWhenUnconnected=off
  FBuf_ext : Outport  Port=4  VectorParamsAs1DForOutWhenUnconnected=off
  wires:
  Bus Creator7/1 -> Terminator4/1
  Bus Creator6/1 -> Terminator3/1
  Bus Creator5/1 -> Terminator2/1
  Bus Creator/1 -> Terminator1/1
  Demux4/8 -> Bus Creator7/8  "vBuf RR"
  Demux4/7 -> Bus Creator7/7  "vBuf RL"
  Demux4/6 -> Bus Creator7/6  "vBuf FR"
  Demux4/5 -> Bus Creator7/5  "vBuf FL"
  Demux3/8 -> Bus Creator6/8  "vStabi RR"
  Demux3/7 -> Bus Creator6/7  "vStabi RL"
  Demux3/6 -> Bus Creator6/6  "vStabi FR"
  Demux3/5 -> Bus Creator6/5  "vStabi FL"
  Demux2/8 -> Bus Creator5/8  "vDamp RR"
  Demux2/7 -> Bus Creator5/7  "vDamp RL"
  Demux2/6 -> Bus Creator5/6  "vDamp FR"
  Demux2/5 -> Bus Creator5/5  "vDamp FL"
  Demux1/8 -> Bus Creator/8  "vSpring RR"
  Demux1/7 -> Bus Creator/7  "vSpring RL"
  Demux1/6 -> Bus Creator/6  "vSpring FR"
  Demux1/5 -> Bus Creator/5  "vSpring FL"
  Demux2/4 -> Bus Creator5/4  "lDamp RR"
  Demux2/3 -> Bus Creator5/3  "lDamp RL"
  Demux2/2 -> Bus Creator5/2  "lDamp FR"
  Demux2/1 -> Bus Creator5/1  "lDamp FL"
  Demux1/4 -> Bus Creator/4  "lSpring RR"
  Demux1/3 -> Bus Creator/3  "lSpring RL"
  Demux1/2 -> Bus Creator/2  "lSpring FR"
  Demux1/1 -> Bus Creator/1  "lSpring FL"
  Demux3/4 -> Bus Creator6/4  "lStabi RR"
  Demux3/3 -> Bus Creator6/3  "lStabi RL"
  Demux3/2 -> Bus Creator6/2  "lStabi FR"
  Demux3/1 -> Bus Creator6/1  "lStabi FL"
  lStabi/1 -> Demux3/1
  vDamp/1 -> Demux2/1
  lSpring/1 -> Demux1/1
  Demux4/4 -> Bus Creator7/4  "lBuf RR"
  Demux4/3 -> Bus Creator7/3  "lBuf RL"
  Demux4/2 -> Bus Creator7/2  "lBuf FR"
  Demux4/1 -> Bus Creator7/1  "lBuf FL"
  lBuf/1 -> Demux4/1
  Ground14/1 -> Bus Creator4/1  "FBuf_ext FL"
  Ground15/1 -> Bus Creator4/2  "FBuf_ext FR"
  Ground12/1 -> Bus Creator4/3  "FBuf_ext RL"
  Ground13/1 -> Bus Creator4/4  "FBuf_ext RR"
  Bus Creator4/1 -> FBuf_ext/1
  Sync_In/1 -> Terminator12/1
  Bus Creator2/1 -> FSpring_ext/1
  Ground/1 -> Bus Creator2/1  "FSpring_ext FL"
  Ground1/1 -> Bus Creator2/2  "FSpring_ext FR"
  Ground2/1 -> Bus Creator2/3  "FSpring_ext RL"
  Ground3/1 -> Bus Creator2/4  "FSpring_ext RR"
  Ground4/1 -> Bus Creator1/1  "FDamp_ext FL"
  Ground5/1 -> Bus Creator1/2  "FDamp_ext FR"
  Ground6/1 -> Bus Creator1/3  "FDamp_ext RL"
  Ground7/1 -> Bus Creator1/4  "FDamp_ext RR"
  Bus Creator1/1 -> FDamp_ext/1
  Ground8/1 -> Bus Creator3/1  "FStabi_ext FL"
  Ground9/1 -> Bus Creator3/2  "FStabi_ext FR"
  Ground10/1 -> Bus Creator3/3  "FStabi_ext RL"
  Ground11/1 -> Bus Creator3/4  "FStabi_ext RR"
  Bus Creator3/1 -> FStabi_ext/1

== system generic_20231123_1032/CarMaker/IPG Vehicle/CarAndTrailer/Forces/Suspension Forces ==
  note: <Your model here>
  note: <Your model here>
  Sync_In : Inport
  lSpring : Inport  Port=2
  vDamp : Inport  Port=3
  lStabi : Inport  Port=4
  lBuf : Inport  Port=5
  Bus Creator{,1..3,8..10} (7 alike) : BusCreator  Inputs=4
  Bus Creator{4..7} (4 alike) : BusCreator  Inputs=6
  Demux{,1..5} (6 alike) : Demux
  Demux{6..9} (4 alike) : Demux  Outputs=6
  Suspension Control Unit : S-Function  FunctionName=CM_Sfun  Parameters='ForcesSuspControl'  SFunctionDeploymentMode=off  EnableBusSupport=off
  Suspension Force Elements : S-Function  FunctionName=CM_Sfun  Parameters='ForcesSusp'  SFunctionDeploymentMode=off  EnableBusSupport=off
  Suspension Force Elements Update : S-Function  FunctionName=CM_Sfun  Parameters='ForcesSuspUpd'  SFunctionDeploymentMode=off  EnableBusSupport=off
  Sync_Out : Outport  VectorParamsAs1DForOutWhenUnconnected=off
  wires:
  vDamp/1 -> Bus Creator8/2
  lStabi/1 -> Bus Creator8/3
  lBuf/1 -> Bus Creator8/4
  lSpring/1 -> Bus Creator8/1
  Bus Creator8/1 -> Suspension Control Unit/2, Suspension Force Elements/2
  Sync_In/1 -> Suspension Control Unit/1
  Suspension Control Unit/1 -> Suspension Force Elements/1
  Suspension Force Elements/1 -> Suspension Force Elements Update/1
  Suspension Force Elements Update/1 -> Sync_Out/1
  Bus Creator4/1 -> Bus Creator10/1
  Bus Creator5/1 -> Bus Creator10/2
  Bus Creator6/1 -> Bus Creator10/3
  Bus Creator7/1 -> Bus Creator10/4
  Demux6/1 -> Bus Creator4/1  "FL SpringForce"
  Demux9/1 -> Bus Creator7/1  "RR SpringForce"
  Demux9/2 -> Bus Creator7/2  "RR DamperForce"
  Demux9/3 -> Bus Creator7/3  "RR StabiForce"
  Demux9/4 -> Bus Creator7/4  "RR BufferForce"
  Demux9/5 -> Bus Creator7/5  "RR ParasiticStiffForce"
  Demux9/6 -> Bus Creator7/6  "RR ParasiticFricForce"
  Demux8/1 -> Bus Creator6/1  "RL SpringForce"
  Demux8/2 -> Bus Creator6/2  "RL DamperForce"
  Demux8/4 -> Bus Creator6/4  "RL BufferForce"
  Demux8/5 -> Bus Creator6/5  "RL ParasiticStiffForce"
  Demux8/6 -> Bus Creator6/6  "RL ParasiticFricForce"
  Demux8/3 -> Bus Creator6/3  "RL StabiForce"
  Demux7/1 -> Bus Creator5/1  "FR SpringForce"
  Demux7/2 -> Bus Creator5/2  "FR DamperForce"
  Demux7/3 -> Bus Creator5/3  "FR StabiForce"
  Demux7/4 -> Bus Creator5/4  "FR BufferForce"
  Demux7/5 -> Bus Creator5/5  "FR ParasiticStiffForce"
  Demux7/6 -> Bus Creator5/6  "FR ParasiticFricForce"
  Demux6/2 -> Bus Creator4/2  "FL DamperForce"
  Demux6/3 -> Bus Creator4/3  "FL StabiForce"
  Demux6/4 -> Bus Creator4/4  "FL BufferForce"
  Demux6/5 -> Bus Creator4/5  "FL ParasiticStiffForce"
  Demux6/6 -> Bus Creator4/6  "FL ParasiticFricForce"
  Bus Creator10/1 -> Suspension Force Elements Update/2
  Demux/1 -> Demux2/1  "FL"
  Bus Creator1/1 -> Bus Creator9/2
  Demux/2 -> Demux3/1  "FR"
  Bus Creator2/1 -> Bus Creator9/3
  Demux/3 -> Demux4/1  "RL"
  Bus Creator3/1 -> Bus Creator9/4
  Demux2/1 -> Bus Creator/1  "FL SpringCtrlOut"
  Demux/4 -> Demux5/1  "RR"
  Demux5/1 -> Bus Creator3/1  "RR SpringCtrlOut"
  Demux5/2 -> Bus Creator3/2  "RR DamperCtrlOut"
  Demux5/3 -> Bus Creator3/3  "RR StabiCtrlOut"
  Demux5/4 -> Bus Creator3/4  "RR BufferCtrlOut"
  Demux4/1 -> Bus Creator2/1  "RL SpringCtrlOut"
  Demux4/2 -> Bus Creator2/2  "RL DamperCtrlOut"
  Demux4/4 -> Bus Creator2/4  "RL BufferCtrlOut"
  Demux4/3 -> Bus Creator2/3  "RL StabiCtrlOut"
  Demux3/1 -> Bus Creator1/1  "FR SpringCtrlOut"
  Demux3/2 -> Bus Creator1/2  "FR DamperCtrlOut"
  Demux3/3 -> Bus Creator1/3  "FR StabiCtrlOut"
  Demux3/4 -> Bus Creator1/4  "FR BufferCtrlOut"
  Demux2/2 -> Bus Creator/2  "FL DamperCtrlOut"
  Demux2/3 -> Bus Creator/3  "FL StabiCtrlOut"
  Demux2/4 -> Bus Creator/4  "FL BufferCtrlOut"
  Suspension Control Unit/2 -> Demux/1
  Bus Creator9/1 -> Suspension Force Elements/3
  Bus Creator/1 -> Bus Creator9/1
  Suspension Force Elements/2 -> Demux1/1
  Demux1/1 -> Demux6/1  "FL"
  Demux1/2 -> Demux7/1  "FR"
  Demux1/3 -> Demux8/1  "RL"
  Demux1/4 -> Demux9/1  "RR"

== system generic_20231123_1032/CarMaker/IPG Vehicle/CarAndTrailer/Forces/Tires ==
  note: The TireXX_Out signals will only be used if FileIdent is "CarMaker-Tire-CM4SL" in the tire parameter file!
      | An example parameter file can be found in Data/Tire/DT_CM4SL_UserTire.
  Sync_In : Inport
  TireFL_In : Inport  Port=2
  TireFR_In : Inport  Port=3
  TireRL_In : Inport  Port=4
  TireRR_In : Inport  Port=5
  Bus Creator{1..4} (4 alike) : BusCreator  Inputs=11
  Demux{1..3,8} (4 alike) : Demux  Outputs=7
      settings: DisplayOption=none
  TireFL : Subsystem
  TireFR : Subsystem
  TireRL : Subsystem
  TireRR : Subsystem
  TireFL_Out : Outport  VectorParamsAs1DForOutWhenUnconnected=off
  TireFR_Out : Outport  Port=2  VectorParamsAs1DForOutWhenUnconnected=off
  TireRL_Out : Outport  Port=3  VectorParamsAs1DForOutWhenUnconnected=off
  TireRR_Out : Outport  Port=4  VectorParamsAs1DForOutWhenUnconnected=off
  wires:
  Sync_In/1 -> TireRR/1(Sync_In), TireRL/1(Sync_In), TireFR/1(Sync_In), TireFL/1(Sync_In)
  Bus Creator4/1 -> TireRR_Out/1
  Bus Creator2/1 -> TireRL_Out/1
  Bus Creator1/1 -> TireFR_Out/1
  Demux3/5 -> TireRR/6(Rim_turnv)  "Tire_In Rim_turnv"
  Demux3/4 -> TireRR/5(Rim_rotv)  "Tire_In Rim_rotv"
  Demux3/1 -> TireRR/2(Load)  "Tire_In Load"
  Demux3/7 -> TireRR/8(muRoad)  "Tire_In mu"
  Demux3/6 -> TireRR/7(InclinAngle)  "Tire_In Camber"
  Demux3/2 -> TireRR/3(vxtrans)  "Tire_In vxtrans"
  Demux3/3 -> TireRR/4(vytrans)  "Tire_In vytrans"
  TireRR/11(AlignTrq) -> Bus Creator4/11  "Tire_Out AlignTrq"
  TireRR/10(RollResist) -> Bus Creator4/10  "Tire_Out RollResist"
  TireRR/9(OverturnTrq) -> Bus Creator4/9  "Tire_Out OverturnTrq"
  TireRR/8(LoadFrc) -> Bus Creator4/8  "Tire_Out LoadFrc"
  TireRR/7(SideFrc) -> Bus Creator4/7  "Tire_Out SideFrc"
  TireRR/6(LongFrc) -> Bus Creator4/6  "Tire_Out LongFrc"
  TireRR/5(vBelt) -> Bus Creator4/5  "Tire_Out vBelt"
  TireRR/4(rBelt_eff) -> Bus Creator4/4  "Tire_Out rBelt_eff"
  TireRR/3(TurnSlp) -> Bus Creator4/3  "Tire_Out TurnSlp"
  TireRR/1(Slp) -> Bus Creator4/1  "Tire_Out Slp"
  TireRR/2(Alpha) -> Bus Creator4/2  "Tire_Out Alpha"
  Demux2/5 -> TireRL/6(Rim_turnv)  "Tire_In Rim_turnv"
  Demux2/4 -> TireRL/5(Rim_rotv)  "Tire_In Rim_rotv"
  Demux2/1 -> TireRL/2(Load)  "Tire_In Load"
  Demux2/7 -> TireRL/8(muRoad)  "Tire_In mu"
  Demux2/6 -> TireRL/7(InclinAngle)  "Tire_In Camber"
  Demux2/2 -> TireRL/3(vxtrans)  "Tire_In vxtrans"
  Demux2/3 -> TireRL/4(vytrans)  "Tire_In vytrans"
  TireRL/11(AlignTrq) -> Bus Creator2/11  "Tire_Out AlignTrq"
  TireRL/10(RollResist) -> Bus Creator2/10  "Tire_Out RollResist"
  TireRL/9(OverturnTrq) -> Bus Creator2/9  "Tire_Out OverturnTrq"
  TireRL/8(LoadFrc) -> Bus Creator2/8  "Tire_Out LoadFrc"
  TireRL/7(SideFrc) -> Bus Creator2/7  "Tire_Out SideFrc"
  TireRL/6(LongFrc) -> Bus Creator2/6  "Tire_Out LongFrc"
  TireRL/5(vBelt) -> Bus Creator2/5  "Tire_Out vBelt"
  TireRL/4(rBelt_eff) -> Bus Creator2/4  "Tire_Out rBelt_eff"
  TireRL/3(TurnSlp) -> Bus Creator2/3  "Tire_Out TurnSlp"
  TireRL/1(Slp) -> Bus Creator2/1  "Tire_Out Slp"
  TireRL/2(Alpha) -> Bus Creator2/2  "Tire_Out Alpha"
  Demux1/5 -> TireFR/6(Rim_turnv)  "Tire_In Rim_turnv"
  Demux1/4 -> TireFR/5(Rim_rotv)  "Tire_In Rim_rotv"
  Demux1/1 -> TireFR/2(Load)  "Tire_In Load"
  Demux1/7 -> TireFR/8(muRoad)  "Tire_In mu"
  Demux1/6 -> TireFR/7(InclinAngle)  "Tire_In Camber"
  Demux1/2 -> TireFR/3(vxtrans)  "Tire_In vxtrans"
  Demux1/3 -> TireFR/4(vytrans)  "Tire_In vytrans"
  TireFR/11(AlignTrq) -> Bus Creator1/11  "Tire_Out AlignTrq"
  TireFR/10(RollResist) -> Bus Creator1/10  "Tire_Out RollResist"
  TireFR/9(OverturnTrq) -> Bus Creator1/9  "Tire_Out OverturnTrq"
  TireFR/8(LoadFrc) -> Bus Creator1/8  "Tire_Out LoadFrc"
  TireFR/7(SideFrc) -> Bus Creator1/7  "Tire_Out SideFrc"
  TireFR/6(LongFrc) -> Bus Creator1/6  "Tire_Out LongFrc"
  TireFR/5(vBelt) -> Bus Creator1/5  "Tire_Out vBelt"
  TireFR/4(rBelt_eff) -> Bus Creator1/4  "Tire_Out rBelt_eff"
  TireFR/3(TurnSlp) -> Bus Creator1/3  "Tire_Out TurnSlp"
  TireFR/1(Slp) -> Bus Creator1/1  "Tire_Out Slp"
  TireFR/2(Alpha) -> Bus Creator1/2  "Tire_Out Alpha"
  Demux8/5 -> TireFL/6(Rim_turnv)  "Tire_In Rim_turnv"
  Demux8/4 -> TireFL/5(Rim_rotv)  "Tire_In Rim_rotv"
  TireFL_In/1 -> Demux8/1
  Demux8/1 -> TireFL/2(Load)  "Tire_In Load"
  Demux8/7 -> TireFL/8(muRoad)  "Tire_In mu"
  Demux8/6 -> TireFL/7(InclinAngle)  "Tire_In Camber"
  Demux8/2 -> TireFL/3(vxtrans)  "Tire_In vxtrans"
  Demux8/3 -> TireFL/4(vytrans)  "Tire_In vytrans"
  TireFL/11(AlignTrq) -> Bus Creator3/11  "Tire_Out AlignTrq"
  TireFL/10(RollResist) -> Bus Creator3/10  "Tire_Out RollResist"
  TireFL/9(OverturnTrq) -> Bus Creator3/9  "Tire_Out OverturnTrq"
  TireFL/8(LoadFrc) -> Bus Creator3/8  "Tire_Out LoadFrc"
  TireFL/7(SideFrc) -> Bus Creator3/7  "Tire_Out SideFrc"
  TireFL/6(LongFrc) -> Bus Creator3/6  "Tire_Out LongFrc"
  TireFL/5(vBelt) -> Bus Creator3/5  "Tire_Out vBelt"
  TireFL/4(rBelt_eff) -> Bus Creator3/4  "Tire_Out rBelt_eff"
  TireFL/3(TurnSlp) -> Bus Creator3/3  "Tire_Out TurnSlp"
  TireFL/1(Slp) -> Bus Creator3/1  "Tire_Out Slp"
  TireFL/2(Alpha) -> Bus Creator3/2  "Tire_Out Alpha"
  Bus Creator3/1 -> TireFL_Out/1
  TireFR_In/1 -> Demux1/1
  TireRL_In/1 -> Demux2/1
  TireRR_In/1 -> Demux3/1
